simulink model "Reactive_System_Accelerator_Pedal_Failure_Model"  (R2024a)
settings: Solver=FixedStepAuto  StartTime=0.0  StopTime=10  RelTol=1e-3
undefined symbols (not defined in the file or in its folder): Reactive_System_Accelerator_Pedal_Failure_Model_Enum
libraries: simulink x5, SignalEditorBlockLib x1
settings Model: Creator=DELL  LastModifiedBy=DELL

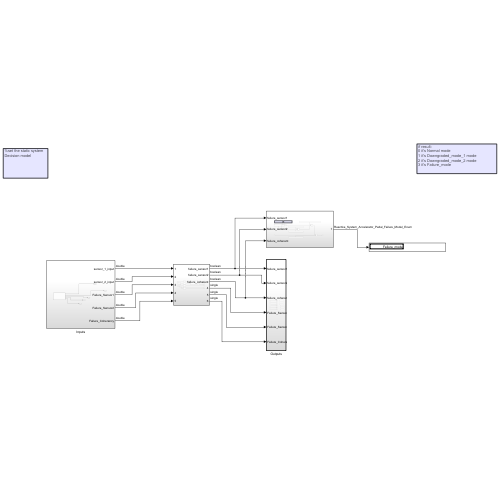
[thumbnail: Simulink's stored preview of the top-level diagram]
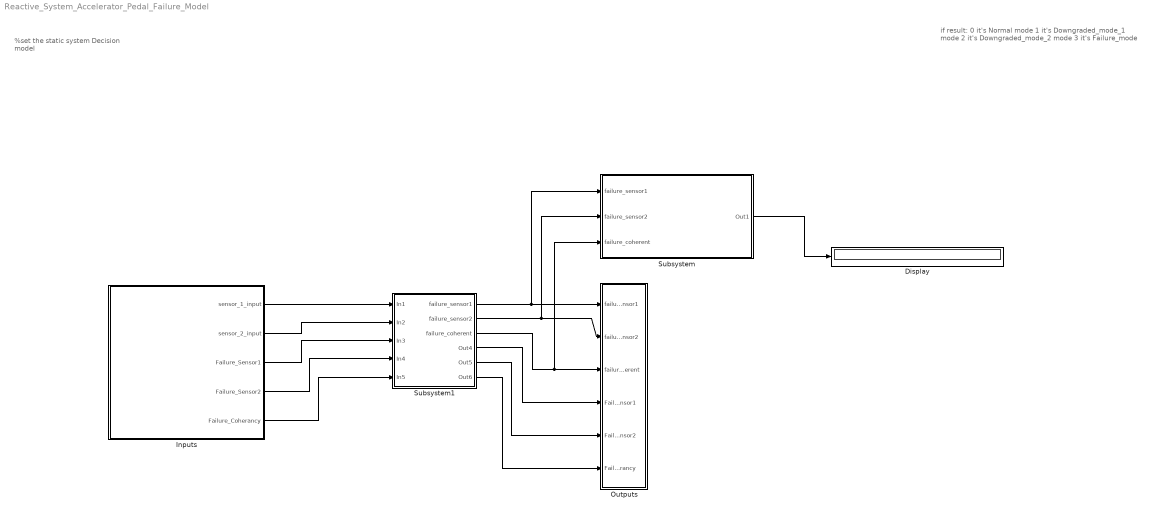
== system Reactive_System_Accelerator_Pedal_Failure_Model ==
  note: %set the static system
      | Decision model
  note: if result:
      | 0 it's Normal mode
      | 1 it's Downgraded_mode_1 mode
      | 2 it's Downgraded_mode_2 mode
      | 3 it's Failure_mode
  Display : Display
  Inputs : Subsystem
  Outputs : Subsystem  TreatAsAtomicUnit=on
  Subsystem : Subsystem
  Subsystem1 : Subsystem
  wires:
  Inputs/1(sensor_1_input) -> Subsystem1/1(In1)
  Inputs/2(sensor_2_input) -> Subsystem1/2(In2)
  Inputs/3(Failure_Sensor1) -> Subsystem1/3(In3)
  Inputs/4(Failure_Sensor2) -> Subsystem1/4(In4)
  Inputs/5(Failure_Coherancy) -> Subsystem1/5(In5)
  Subsystem1/2(failure_sensor2) -> Subsystem/2(failure_sensor2), Outputs/2(failure_sensor2)
  Subsystem1/3(failure_coherent) -> Subsystem/3(failure_coherent), Outputs/3(failure_coherent)
  Subsystem1/4(Out4) -> Outputs/4(Failure_Sensor1)
  Subsystem1/5(Out5) -> Outputs/5(Failure_Sensor2)
  Subsystem1/6(Out6) -> Outputs/6(Failure_Coherancy)
  Subsystem1/1(failure_sensor1) -> Subsystem/1(failure_sensor1), Outputs/1(failure_sensor1)
  Subsystem/1(Out1) -> Display/1

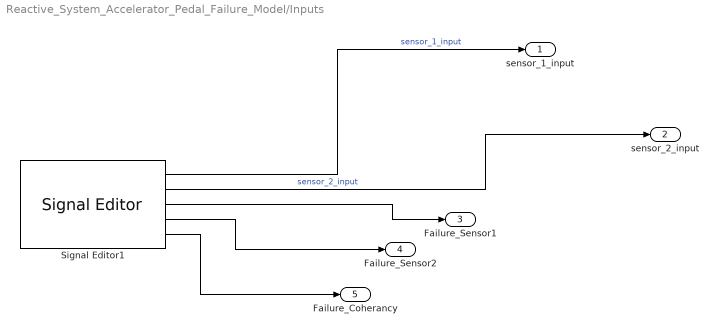
== system Reactive_System_Accelerator_Pedal_Failure_Model/Inputs ==
  Signal Editor1 : SignalEditorBlockLib/Signal Editor  FileName=Test_TPS.mat  ActiveScenario=Sheet2  ActiveSignal=TPS_Sensor1_Voltage  IsBus=off  OutputBusObjectStr=Bus: BusObject  SampleTime=0  Interpolate=off  ZeroCross=off  OutputAfterFinalValue=Setting to zero  Unit=inherit  PreserveSignalName=on  ApplySigPropsToAllScenarios=on  ApplySigPropsToAllSignals=off
  sensor_1_input : Outport
  sensor_2_input : Outport  Port=2
  Failure_Sensor1 : Outport  Port=3
  Failure_Sensor2 : Outport  Port=4
  Failure_Coherancy : Outport  Port=5
  wires:
  Signal Editor1/2 -> sensor_2_input/1  "sensor_2_input"
  Signal Editor1/1 -> sensor_1_input/1  "sensor_1_input"
  Signal Editor1/5 -> Failure_Coherancy/1
  Signal Editor1/3 -> Failure_Sensor1/1
  Signal Editor1/4 -> Failure_Sensor2/1

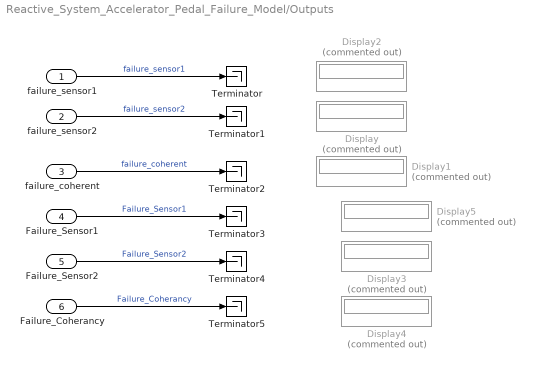
== system Reactive_System_Accelerator_Pedal_Failure_Model/Outputs ==
  failure_sensor1 : Inport
  failure_sensor2 : Inport  Port=2
  failure_coherent : Inport  Port=3
  Failure_Sensor1 : Inport  Port=4
  Failure_Sensor2 : Inport  Port=5
  Failure_Coherancy : Inport  Port=6
  Display{,1..5} (6 alike) : Display  Commented=on
  Terminator{,1..5} (6 alike) : Terminator
  wires:
  failure_sensor2/1 -> Terminator1/1  "failure_sensor2"
  failure_sensor1/1 -> Terminator/1  "failure_sensor1"
  failure_coherent/1 -> Terminator2/1  "failure_coherent"
  Failure_Sensor1/1 -> Terminator3/1  "Failure_Sensor1"
  Failure_Coherancy/1 -> Terminator5/1  "Failure_Coherancy"
  Failure_Sensor2/1 -> Terminator4/1  "Failure_Sensor2"

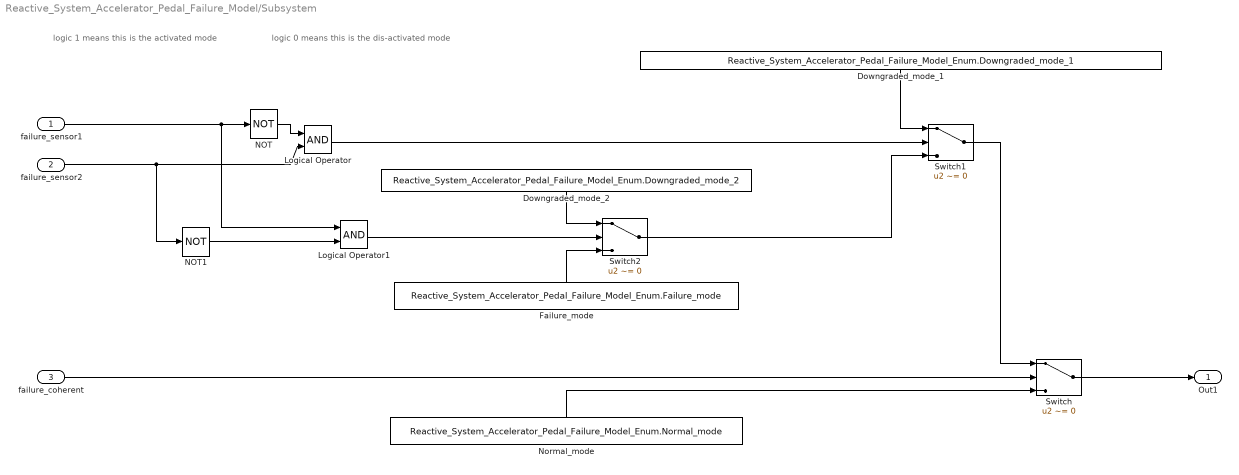
== system Reactive_System_Accelerator_Pedal_Failure_Model/Subsystem ==
  note: logic 1
      | means this is the activated mode
  note: logic 0
      | means this is the dis-activated mode
  failure_sensor1 : Inport
  failure_sensor2 : Inport  Port=2
  failure_coherent : Inport  Port=3
  Downgraded_mode_1 : Constant  Value=Reactive_System_Accelerator_Pedal_Failure_Model_Enum.Downgraded_mode_1
  Downgraded_mode_2 : Constant  Value=Reactive_System_Accelerator_Pedal_Failure_Model_Enum.Downgraded_mode_2
  Failure_mode : Constant  Value=Reactive_System_Accelerator_Pedal_Failure_Model_Enum.Failure_mode
  Logical Operator : Logic  AllPortsSameDT=off  OutDataTypeStr=boolean
  Logical Operator1 : Logic  AllPortsSameDT=off  OutDataTypeStr=boolean
  NOT : Logic  Operator=NOT  IconShape=distinctive  AllPortsSameDT=off  OutDataTypeStr=boolean
  NOT1 : Logic  Operator=NOT  IconShape=distinctive  AllPortsSameDT=off  OutDataTypeStr=boolean
  Normal_mode : Constant  Value=Reactive_System_Accelerator_Pedal_Failure_Model_Enum.Normal_mode
  Switch : Switch  Criteria=u2 ~= 0  SaturateOnIntegerOverflow=off  InputSameDT=off
  Switch1 : Switch  Criteria=u2 ~= 0  SaturateOnIntegerOverflow=off  InputSameDT=off
  Switch2 : Switch  Criteria=u2 ~= 0  SaturateOnIntegerOverflow=off  InputSameDT=off
  Out1 : Outport
  wires:
  failure_coherent/1 -> Switch/2
  Normal_mode/1 -> Switch/3
  failure_sensor1/1 -> NOT/1, Logical Operator1/1
  NOT/1 -> Logical Operator/1
  failure_sensor2/1 -> Logical Operator/2, NOT1/1
  NOT1/1 -> Logical Operator1/2
  Logical Operator/1 -> Switch1/2
  Downgraded_mode_1/1 -> Switch1/1
  Logical Operator1/1 -> Switch2/2
  Downgraded_mode_2/1 -> Switch2/1
  Failure_mode/1 -> Switch2/3
  Switch2/1 -> Switch1/3
  Switch1/1 -> Switch/1
  Switch/1 -> Out1/1

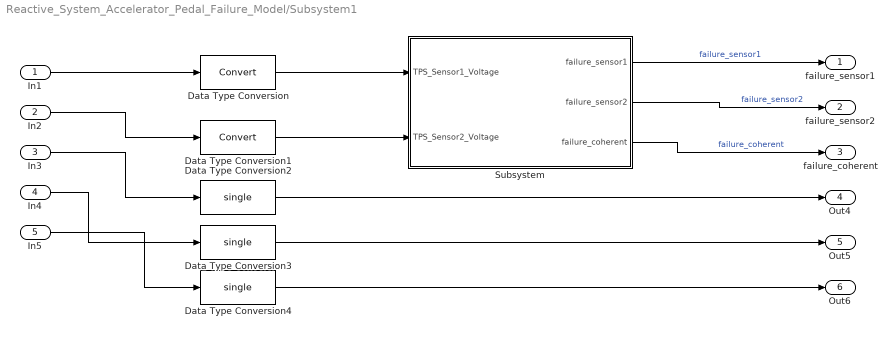
== system Reactive_System_Accelerator_Pedal_Failure_Model/Subsystem1 ==
  In1 : Inport
  In2 : Inport  Port=2
  In3 : Inport  Port=3
  In4 : Inport  Port=4
  In5 : Inport  Port=5
  Data Type Conversion : DataTypeConversion  SaturateOnIntegerOverflow=off  RndMeth=Floor
  Data Type Conversion1 : DataTypeConversion  SaturateOnIntegerOverflow=off  RndMeth=Floor
  Data Type Conversion2 : DataTypeConversion  OutDataTypeStr=single  SaturateOnIntegerOverflow=off  RndMeth=Floor
  Data Type Conversion3 : DataTypeConversion  OutDataTypeStr=single  SaturateOnIntegerOverflow=off  RndMeth=Floor
  Data Type Conversion4 : DataTypeConversion  OutDataTypeStr=single  SaturateOnIntegerOverflow=off  RndMeth=Floor
  Subsystem : Subsystem  TreatAsAtomicUnit=on
  failure_sensor1 : Outport
  failure_sensor2 : Outport  Port=2
  failure_coherent : Outport  Port=3
  Out4 : Outport  Port=4
  Out5 : Outport  Port=5
  Out6 : Outport  Port=6
  wires:
  Data Type Conversion1/1 -> Subsystem/2(TPS_Sensor2_Voltage)
  In5/1 -> Data Type Conversion4/1
  Subsystem/1(failure_sensor1) -> failure_sensor1/1  "failure_sensor1"
  Data Type Conversion/1 -> Subsystem/1(TPS_Sensor1_Voltage)
  Subsystem/2(failure_sensor2) -> failure_sensor2/1  "failure_sensor2"
  Data Type Conversion4/1 -> Out6/1
  Data Type Conversion2/1 -> Out4/1
  In3/1 -> Data Type Conversion2/1
  Data Type Conversion3/1 -> Out5/1
  In2/1 -> Data Type Conversion1/1
  Subsystem/3(failure_coherent) -> failure_coherent/1  "failure_coherent"
  In4/1 -> Data Type Conversion3/1
  In1/1 -> Data Type Conversion/1

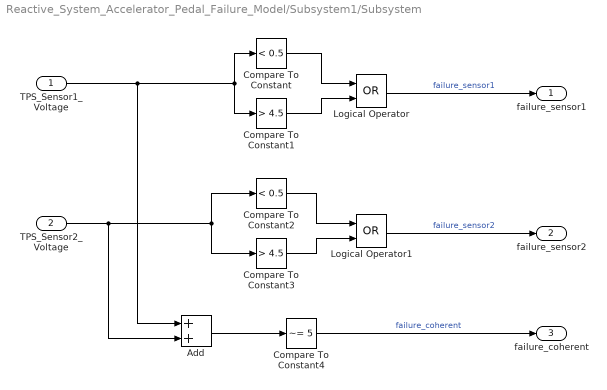
== system Reactive_System_Accelerator_Pedal_Failure_Model/Subsystem1/Subsystem ==
  TPS_Sensor1_Voltage : Inport  OutDataTypeStr=single
  TPS_Sensor2_Voltage : Inport  Port=2  OutDataTypeStr=single
  Add : Sum
  Compare To Constant : simulink/Logic and Bit Operations/Compare To Constant  relop=<  const=0.5  OutDataTypeStr=boolean
  Compare To Constant1 : simulink/Logic and Bit Operations/Compare To Constant  relop=>  const=4.5  OutDataTypeStr=boolean
  Compare To Constant2 : simulink/Logic and Bit Operations/Compare To Constant  relop=<  const=0.5  OutDataTypeStr=boolean
  Compare To Constant3 : simulink/Logic and Bit Operations/Compare To Constant  relop=>  const=4.5  OutDataTypeStr=boolean  ZeroCross=off
  Compare To Constant4 : simulink/Logic and Bit Operations/Compare To Constant  relop=~=  const=5  OutDataTypeStr=boolean
  Logical Operator : Logic  Operator=OR  AllPortsSameDT=off  OutDataTypeStr=boolean
  Logical Operator1 : Logic  Operator=OR  AllPortsSameDT=off  OutDataTypeStr=boolean
  failure_sensor1 : Outport  OutDataTypeStr=boolean
  failure_sensor2 : Outport  Port=2  OutDataTypeStr=boolean
  failure_coherent : Outport  Port=3  OutDataTypeStr=boolean
  wires:
  Compare To Constant/1 -> Logical Operator/1
  Compare To Constant1/1 -> Logical Operator/2
  Logical Operator/1 -> failure_sensor1/1  "failure_sensor1"
  TPS_Sensor1_Voltage/1 -> Add/1, Compare To Constant/1, Compare To Constant1/1
  TPS_Sensor2_Voltage/1 -> Add/2, Compare To Constant3/1, Compare To Constant2/1
  Compare To Constant2/1 -> Logical Operator1/1
  Compare To Constant3/1 -> Logical Operator1/2
  Logical Operator1/1 -> failure_sensor2/1  "failure_sensor2"
  Add/1 -> Compare To Constant4/1
  Compare To Constant4/1 -> failure_coherent/1  "failure_coherent"
